simulink library "dgi"  (Simulink 8.2)
settings: Solver=ode45  SolverMode=SingleTasking  StartTime=0.0  StopTime=10.0  RelTol=1e-3
settings Model: Creator=13192  LastModifiedBy=13192

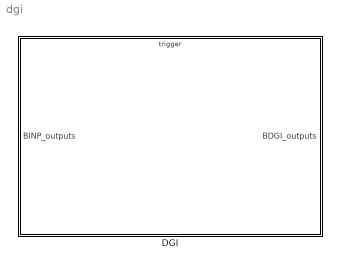
== system dgi ==
  DGI : Subsystem
      settings: RTWSystemCode=Nonreusable function  RTWFcnNameOpts=Use subsystem name  RTWFileNameOpts=Use subsystem name

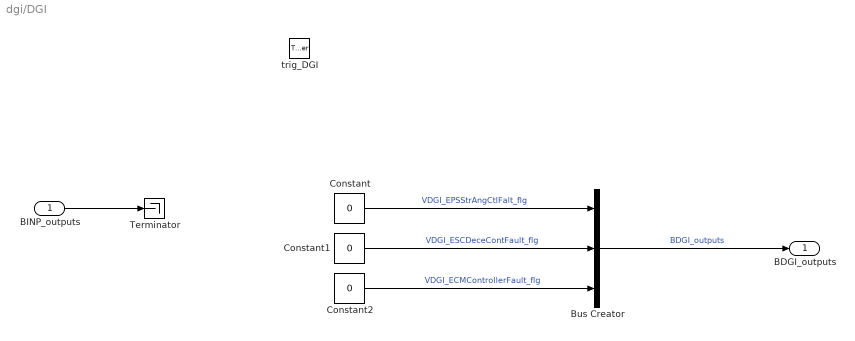
== system dgi/DGI ==
  BINP_outputs : Inport  OutDataTypeStr=Bus: BINP_outputs
  trig_DGI : TriggerPort  TriggerType=function-call
  Bus Creator : BusCreator  Inputs=3  OutDataTypeStr=Bus: BDGI_outputs
  Constant : Constant  Value=0  OutDataTypeStr=boolean
  Constant1 : Constant  Value=0  OutDataTypeStr=boolean
  Constant2 : Constant  Value=0  OutDataTypeStr=boolean
  Terminator : Terminator
  BDGI_outputs : Outport  OutDataTypeStr=Bus: BDGI_outputs
  wires:
  Bus Creator/1 -> BDGI_outputs/1  "BDGI_outputs"
  Constant/1 -> Bus Creator/1  "VDGI_EPSStrAngCtlFalt_flg"
  BINP_outputs/1 -> Terminator/1
  Constant1/1 -> Bus Creator/2  "VDGI_ESCDeceContFault_flg"
  Constant2/1 -> Bus Creator/3  "VDGI_ECMControllerFault_flg"
